simulink model "LAB4T3"  (R2018b)
settings: Solver=VariableStepAuto  StartTime=0.0  StopTime=10.0  RelTol=1e-3
settings Model: Creator=aloisia  LastModifiedBy=aloisia

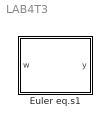
== system LAB4T3 ==
  Euler eq.s1 : MATLAB Function  TreatAsAtomicUnit=on

== matlab function LAB4T3/Euler eq.s1 ==
  data: w input; y output
function y = euler_eqs(w)

J1=0.01;
J2=0.1;
J3=0.07;

w_dot = zeros(3,1);

c1 = ((J2-J3)/J1);
c2 = ((J3-J1)/J2);
c3 = ((J1-J2)/J3);

w_dot(1) = c1*w(2)*w(3);
w_dot(2) = c2*w(1)*w(3) ;
w_dot(3) = c3*w(2)*w(1);

y=w_dot;
